simulink model "d_4_dc_motor_bar"  (R2014b)
settings: Solver=ode45  StartTime=0.0  StopTime=100  RelTol=1e-3
values from neighbouring files (symbols this model uses):
  Bm = 0.01    [d_1_dc_motor_parameter.m]    (also in d_2_draw_wt_theta_real.m; d_2_draw_wt_theta_tf.m; d_4_dc_motor_bar_parameter.m; plot.m)
  g = 9.8    [d_4_dc_motor_bar_parameter.m]    (also in tham_so.m)
  Jm = 0.000052    (= 5.2e-05)    [d_1_dc_motor_parameter.m]    (also in d_2_draw_wt_theta_real.m; d_2_draw_wt_theta_tf.m; d_4_dc_motor_bar_parameter.m; plot.m)
  Ke = 0.235    [d_1_dc_motor_parameter.m]    (also in d_2_draw_wt_theta_real.m; d_2_draw_wt_theta_tf.m; d_4_dc_motor_bar_parameter.m; plot.m)
  Kt = 0.235    [d_1_dc_motor_parameter.m]    (also in d_2_draw_wt_theta_real.m; d_2_draw_wt_theta_tf.m; d_4_dc_motor_bar_parameter.m; plot.m)
  La = 0.23    [d_1_dc_motor_parameter.m]    (also in d_2_draw_wt_theta_real.m; d_2_draw_wt_theta_tf.m; d_4_dc_motor_bar_parameter.m; plot.m)
  m_bar = 0    [d_4_dc_motor_bar_parameter.m]    (also in tham_so.m)
  Ra = 2    [d_1_dc_motor_parameter.m]    (also in d_2_draw_wt_theta_real.m; d_2_draw_wt_theta_tf.m; d_4_dc_motor_bar_parameter.m; plot.m)
libraries: simulink x2
settings Model: Creator=Admin  LastModifiedBy=Admin

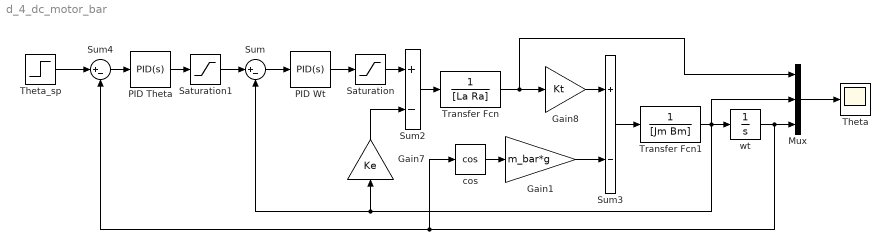
== system d_4_dc_motor_bar ==
  Gain1 : Gain  Gain=m_bar*g
  Gain7 : Gain  Gain=Ke
  Gain8 : Gain  Gain=Kt
  Mux : Mux  Inputs=3
  PID Theta : simulink/Continuous/PID Controller  Controller=PID  TimeDomain=Continuous-time  SampleTime=-1  IntegratorMethod=Forward Euler  FilterMethod=Forward Euler  Form=Parallel  P=1  I=0  D=0  N=0  InitialConditionSource=internal  InitialConditionForIntegrator=0  InitialConditionForFilter=0  ExternalReset=none  LimitOutput=off  UpperSaturationLimit=inf  LowerSaturationLimit=-inf  LinearizeAsGain=on  AntiWindupMode=none  Kb=1  TrackingMode=off  Kt=1  PParamMin=[]  PParamMax=[]  IParamMin=[]  IParamMax=[]  DParamMin=[]  DParamMax=[]  NParamMin=[]  NParamMax=[]  KbParamMin=[]  KbParamMax=[]  KtParamMin=[]  KtParamMax=[]  POutMin=[]  POutMax=[]  IOutMin=[]  IOutMax=[]  DOutMin=[]  DOutMax=[]  NOutMin=[]  NOutMax=[]  KbOutMin=[]  KbOutMax=[]  KtOutMin=[]  KtOutMax=[]  IntegratorOutMin=[]  IntegratorOutMax=[]  FilterOutMin=[]  FilterOutMax=[]  SumOutMin=[]  SumOutMax=[]  SumI1OutMin=[]  SumI1OutMax=[]  SumI2OutMin=[]  SumI2OutMax=[]  SumI3OutMin=[]  SumI3OutMax=[]  SumDOutMin=[]  SumDOutMax=[]  SaturationOutMin=[]  SaturationOutMax=[]  IntegratorContinuousStateAttributes=''  IntegratorStateMustResolveToSignalObject=off  IntegratorRTWStateStorageClass=Auto  FilterContinuousStateAttributes=''  FilterStateMustResolveToSignalObject=off  FilterRTWStateStorageClass=Auto  DifferentiatorICPrevScaledInput=0  DifferentiatorOutMin=[]  DifferentiatorOutMax=[]  UseFilter=on
  PID Wt : simulink/Continuous/PID Controller  Controller=PID  TimeDomain=Continuous-time  SampleTime=-1  IntegratorMethod=Forward Euler  FilterMethod=Forward Euler  Form=Parallel  P=0.1  I=0.5  D=0  N=0  InitialConditionSource=internal  InitialConditionForIntegrator=0  InitialConditionForFilter=0  ExternalReset=none  LimitOutput=off  UpperSaturationLimit=inf  LowerSaturationLimit=-inf  LinearizeAsGain=on  AntiWindupMode=none  Kb=1  TrackingMode=off  Kt=1  PParamMin=[]  PParamMax=[]  IParamMin=[]  IParamMax=[]  DParamMin=[]  DParamMax=[]  NParamMin=[]  NParamMax=[]  KbParamMin=[]  KbParamMax=[]  KtParamMin=[]  KtParamMax=[]  POutMin=[]  POutMax=[]  IOutMin=[]  IOutMax=[]  DOutMin=[]  DOutMax=[]  NOutMin=[]  NOutMax=[]  KbOutMin=[]  KbOutMax=[]  KtOutMin=[]  KtOutMax=[]  IntegratorOutMin=[]  IntegratorOutMax=[]  FilterOutMin=[]  FilterOutMax=[]  SumOutMin=[]  SumOutMax=[]  SumI1OutMin=[]  SumI1OutMax=[]  SumI2OutMin=[]  SumI2OutMax=[]  SumI3OutMin=[]  SumI3OutMax=[]  SumDOutMin=[]  SumDOutMax=[]  SaturationOutMin=[]  SaturationOutMax=[]  IntegratorContinuousStateAttributes=''  IntegratorStateMustResolveToSignalObject=off  IntegratorRTWStateStorageClass=Auto  FilterContinuousStateAttributes=''  FilterStateMustResolveToSignalObject=off  FilterRTWStateStorageClass=Auto  DifferentiatorICPrevScaledInput=0  DifferentiatorOutMin=[]  DifferentiatorOutMax=[]  UseFilter=on
  Saturation : Saturate  UpperLimit=24  LowerLimit=-24
  Saturation1 : Saturate  UpperLimit=74  LowerLimit=-74
  Sum : Sum  Inputs=|+-
  Sum2 : Sum  Inputs=+-
  Sum3 : Sum  Inputs=+-
  Sum4 : Sum  Inputs=|+-
  Theta : Scope
      settings: TimeRange=1  YMin=-1  YMax=1  SaveName=ScopeData4
  Theta_sp : Step  Time=0  After=10  SampleTime=0
  Transfer Fcn : TransferFcn  Denominator=[La Ra]
  Transfer Fcn1 : TransferFcn  Denominator=[Jm Bm]
  cos : Trigonometry  Operator=cos
  wt : Integrator
  wires:
  Sum/1 -> PID Wt/1
  Gain7/1 -> Sum2/2
  Gain8/1 -> Sum3/1
  Transfer Fcn/1 -> Mux/1, Gain8/1
  PID Wt/1 -> Saturation/1
  Sum3/1 -> Transfer Fcn1/1
  Transfer Fcn1/1 -> Mux/2, wt/1, Sum/2, Gain7/1
  wt/1 -> Mux/3, Sum4/2, cos/1
  Sum2/1 -> Transfer Fcn/1
  Sum4/1 -> PID Theta/1
  Theta_sp/1 -> Sum4/1
  PID Theta/1 -> Saturation1/1
  Mux/1 -> Theta/1
  Saturation/1 -> Sum2/1
  Saturation1/1 -> Sum/1
  Gain1/1 -> Sum3/2
  cos/1 -> Gain1/1
